simulink model "oscillator1"  (R2018b)
settings: Solver=FixedStepAuto  StartTime=0.0  StopTime=40  FixedStep=0.001  RelTol=1e-3
settings Model: Creator=User  LastModifiedBy=User

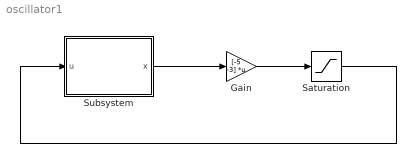
== system oscillator1 ==
  Gain : Gain  Gain=[-5 -3]  Multiplication=Matrix(K*u)
  Saturation : Saturate  UpperLimit=1  LowerLimit=-1
  Subsystem : Subsystem
  wires:
  Subsystem/1(x) -> Gain/1
  Gain/1 -> Saturation/1
  Saturation/1 -> Subsystem/1(u)

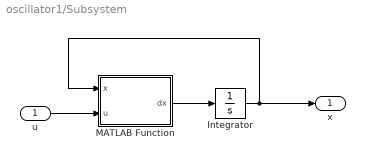
== system oscillator1/Subsystem ==
  u : Inport
  Integrator : Integrator  InitialCondition=[0;1]
  MATLAB Function : MATLAB Function  TreatAsAtomicUnit=on
  x : Outport
  wires:
  Integrator/1 -> x/1, MATLAB Function/1(x)
  MATLAB Function/1(dx) -> Integrator/1
  u/1 -> MATLAB Function/2(u)

== matlab function oscillator1/Subsystem/MATLAB Function ==
  data: x input; u input; dx output
function dx = fcn(x,u)
x1=x(1);
x2=x(2);
dx=[x1+x2-x1*(x1^2+x2^2);
    -x1+x2-x2*(x1^2+x2^2)+u];
end
